simulink model "cnlib"  (Simulink 6.2)
settings: Solver=ode5  SolverMode=SingleTasking  StartTime=0.0  StopTime=5  FixedStep=0.001  MaxStep=0.001  RelTol=1e-3  AbsTol=1e-3
undefined symbols (not defined in the file): k
(part 1 of 7)
settings Model: Creator=jacobs  LastModifiedBy=jacobs  ExtModeAutoUpdateStatusClock=off
settings DataIOCC: LimitDataPoints=off  SaveOutput=off  SaveTime=off
settings OptimizationCC: BlockReduction=off  BooleanDataType=off
settings HardwareCC: TargetUnknown=on
settings STFCustomTargetCC: TargetFcnLib=ansi_tfl_tmw.mat  GenFloatMathFcnCalls=ANSI_C  ModelReferenceCompliant=off  SystemTargetFile=grt.tlc

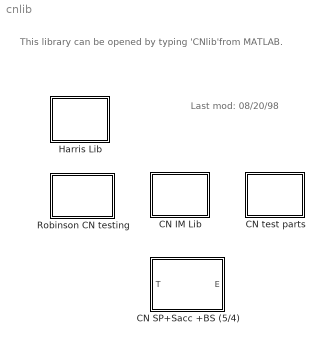
== system cnlib ==
  note: This library can be opened by typing
      |  'CNlib'from MATLAB.
  note: Last mod:
      | 08/20/98
  CN IM Lib : Subsystem
      mask Type: Lib
      mask Display: disp('CN IM\nLib')
  CN SP+Sacc +BS (5/4) : Subsystem
      mask init:
      | k=0.25;
      mask Display: disp('CN Model\nSP (DARm)\nSacc+BS')
  CN test parts : Subsystem
      mask Type: Lib
      mask Display: disp('CN Test\nParts')
  Harris Lib : Subsystem
      mask Display: disp('Harris\nLibrary')
  Robinson CN testing : Subsystem
      mask Display: disp('Robinson\nCN test')

== system cnlib/CN IM Lib ==
  BS Logic1 : Subsystem  Orientation=up
      mask Display: disp('BS/FS\nLogic')
  FS or BS? : Subsystem
      mask Display: disp('FS/BS?')
  IM (SP) 1z2p : Subsystem
      mask Display: disp('IM (SP)')
  IM (SP) 2p : Subsystem
      mask Display: disp('IM (SP)')
  IM (sacc) (FS) (old) : Subsystem
      mask Display: disp('IM (Sacc)')
  IM (sacc) (FS+BS) (old) : Subsystem
      mask Display: disp('IM (Sacc)')
  "IM (sacc) (FS+BS) (old) " : Subsystem
      mask Display: disp('IM (Sacc)')
  IM (sp) 1p : Subsystem
      mask Display: disp('IM (SP)')
  IM SP + Sacc (pos-vel) : Subsystem  Orientation=left
      mask Display: disp('IM\nSP + Sacc\n(pos-vel)')
  IM Sacc (pos-vel) (good!) : Subsystem
      mask Display: disp('IM\nSP + Sacc\n(pos-vel)')

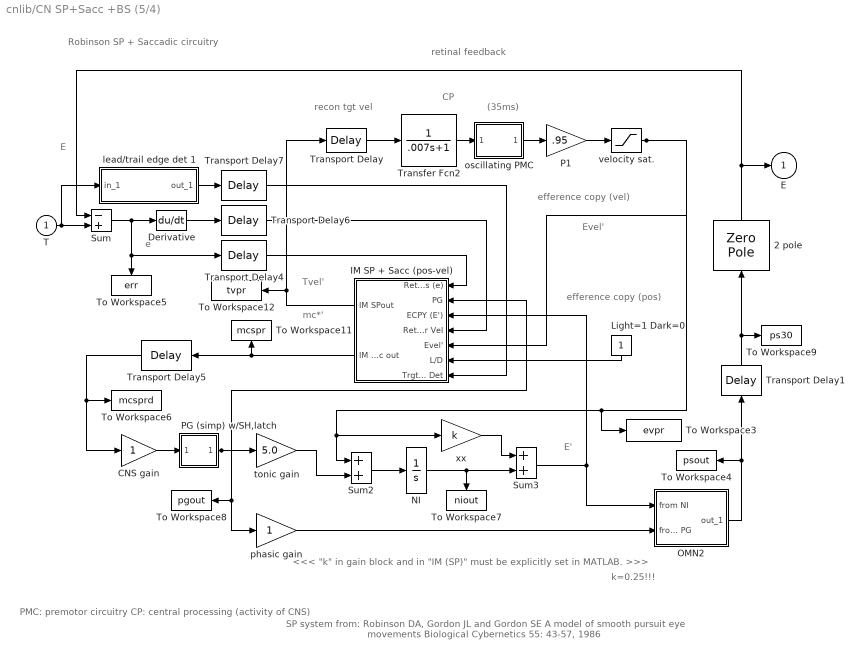
== system cnlib/CN SP+Sacc +BS (5/4) ==
  note: efference copy (pos)
  note: Evel'
  note: mc*'
  note: Tvel'
  note: e
  note: E
  note: E'
  note: k=0.25!!!
  note: retinal feedback
  note: recon tgt vel
  note: efference copy (vel)
  note: CP
  note: <<<  "k" in gain block and in "IM (SP)"
      | must be explicitly set in MATLAB.  >>>
  note: Robinson SP + Saccadic circuitry
  note: PMC: premotor circuitry
      | CP: central processing (activity of CNS)
  note: SP system from: Robinson DA, Gordon JL and Gordon SE
      | A model of smooth pursuit eye movements
      | Biological Cybernetics 55: 43-57,  1986
  note: (35ms)
  T : Inport  Port=1  LatchInput=off
  2 pole : ZeroPole  Orientation=up  Zeros=[ ]  Poles=[ -1/.18 -1/.007]  Gain=[1/.18 * 1/.007]
      mask Display: disp('2-pole\nPlant')
  CNS gain : Gain  SaturateOnIntegerOverflow=on
  Derivative : Derivative
      mask Display: disp('s')
  IM SP + Sacc (pos-vel) : Subsystem  Orientation=left
      mask Display: disp('IM\nSP + Sacc\n(pos-vel)')
  Light=1 Dark=0 : Constant  Orientation=down
  NI : Integrator
  OMN2 : Subsystem
      mask Display: disp('<--"tonic" \nOMN2\n<--"phasic"')
  P1 : Gain  Gain=.95  SaturateOnIntegerOverflow=on
  PG (simp) w/SH,latch : Subsystem
      mask Display: disp('PG')
  Sum : Sum  Inputs=-+  SaturateOnIntegerOverflow=on  InputSameDT=on
  Sum2 : Sum  SaturateOnIntegerOverflow=on  InputSameDT=on
  Sum3 : Sum  SaturateOnIntegerOverflow=on  InputSameDT=on
  To Workspace11 : ToWorkspace  VariableName=mcspr  SaveFormat=Array
      settings: Orientation=up  MaxDataPoints=10000
  To Workspace12 : ToWorkspace  VariableName=tvpr  SaveFormat=Array
      settings: MaxDataPoints=10000
  To Workspace3 : ToWorkspace  VariableName=evpr  SaveFormat=Array
      settings: MaxDataPoints=10000
  To Workspace4 : ToWorkspace  VariableName=psout  SaveFormat=Array
      settings: MaxDataPoints=10000
  To Workspace5 : ToWorkspace  VariableName=err  SaveFormat=Array
      settings: Orientation=down  MaxDataPoints=10000
  To Workspace6 : ToWorkspace  VariableName=mcsprd  SaveFormat=Array
      settings: MaxDataPoints=10000
  To Workspace7 : ToWorkspace  VariableName=niout  SaveFormat=Array
      settings: Orientation=down  MaxDataPoints=10000
  To Workspace8 : ToWorkspace  VariableName=pgout  SaveFormat=Array
      settings: MaxDataPoints=10000
  To Workspace9 : ToWorkspace  VariableName=ps30  SaveFormat=Array
      settings: MaxDataPoints=10000
  Transfer Fcn2 : TransferFcn  Denominator=[.007 1]
  Transport Delay : TransportDelay  DelayTime=0.015
      mask Display: disp('15ms')
  Transport Delay1 : TransportDelay  Orientation=up  DelayTime=0.03
      mask Display: disp('30ms')
  Transport Delay4 : TransportDelay  DelayTime=.05
      mask Display: disp('50ms')
  Transport Delay5 : TransportDelay  Orientation=left  DelayTime=0.001
      mask Display: disp('1ms')
  Transport Delay6 : TransportDelay  DelayTime=.05
      mask Display: disp('50ms')
  Transport Delay7 : TransportDelay  DelayTime=.05
      mask Display: disp('50ms')
  lead/trail edge det 1 : Subsystem
      mask Display: disp('Target Change\nDetection')
  oscillating PMC : Subsystem
      mask Display: disp('PMC+')
  phasic gain : Gain  SaturateOnIntegerOverflow=on
  tonic gain : Gain  Gain=5.0  SaturateOnIntegerOverflow=on
  velocity sat. : Saturate  UpperLimit=90  LowerLimit=-90
  xx : Gain  Gain=k  SaturateOnIntegerOverflow=on
  E : Outport  InitialOutput=0
  wires:
  Transport Delay5/1 -> CNS gain/1, To Workspace6/1
  CNS gain/1 -> PG (simp) w/SH,latch/1(in_1)
  PG (simp) w/SH,latch/1(out_1) -> phasic gain/1, To Workspace8/1, IM SP + Sacc (pos-vel)/2(PG), tonic gain/1
  IM SP + Sacc (pos-vel)/2(IM Sacc out) -> Transport Delay5/1, To Workspace11/1
  Transport Delay7/1 -> IM SP + Sacc (pos-vel)/7(TrgtChng Det)
  lead/trail edge det 1/1(out_1) -> Transport Delay7/1
  IM SP + Sacc (pos-vel)/1(IM SPout) -> Transport Delay/1, To Workspace12/1
  Derivative/1 -> Transport Delay6/1
  Transport Delay6/1 -> IM SP + Sacc (pos-vel)/4(RetErr Vel)
  Transport Delay1/1 -> 2 pole/1, To Workspace9/1
  Sum/1 -> Derivative/1, Transport Delay4/1, To Workspace5/1
  NI/1 -> Sum3/2, To Workspace7/1
  Sum3/1 -> IM SP + Sacc (pos-vel)/3(ECPY (E')), OMN2/1(from NI)
  velocity sat./1 -> IM SP + Sacc (pos-vel)/5(Evel'), Sum2/1, xx/1, To Workspace3/1
  Light=1 Dark=0/1 -> IM SP + Sacc (pos-vel)/6(L/D)
  xx/1 -> Sum3/1
  2 pole/1 -> E/1, Sum/1
  phasic gain/1 -> OMN2/2(from PG)
  OMN2/1(out_1) -> Transport Delay1/1, To Workspace4/1
  T/1 -> lead/trail edge det 1/1(in_1), Sum/2
  Sum2/1 -> NI/1
  tonic gain/1 -> Sum2/2
  Transfer Fcn2/1 -> oscillating PMC/1(desired eye vel)
  P1/1 -> velocity sat./1
  oscillating PMC/1(efference copy eye vel) -> P1/1
  Transport Delay/1 -> Transfer Fcn2/1
  Transport Delay4/1 -> IM SP + Sacc (pos-vel)/1(RetErr Pos (e))

== system cnlib/CN test parts ==
  Tgt moved? : Subsystem
      mask Display: disp('Tgt\nmoved?')
  mult sacc test : Subsystem
      mask Display: disp('mult\nsacc\ntest')
  summing test : Subsystem

== system cnlib/Harris Lib ==
  note: Harris Lib
  Harris Model : Subsystem
      mask Display: disp('Harris\n''95')

== system cnlib/Robinson CN testing ==
  note: Robinson Library (CN Testing)
  note: Last mod:
      | 08/20/98
  Robinson Fig. 8' : Subsystem
      mask Display: disp('Robinson\n(Osc.)')
  accel saturation : MATLABFcn  MATLABFcn=accsat
      mask Display: plot([-40 -8 8 40],[-120 -60 60 120], [0 0],[-120 120],[-40 40],[0 0])
  original PMC : Subsystem
      mask Display: disp('PMC')
  oscillating PMC : Subsystem
      mask Display: disp('PMC+')

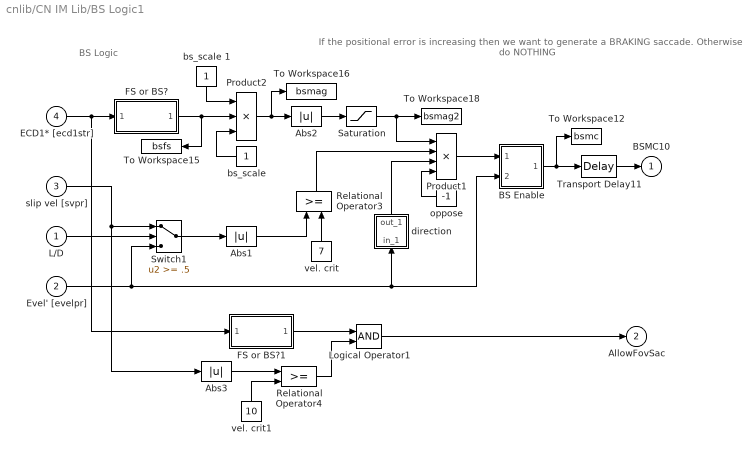
== system cnlib/CN IM Lib/BS Logic1 ==
  note: If the positional error is increasing then we want
      | to generate a BRAKING saccade.  Otherwise do NOTHING
  note: BS Logic
  L/D : Inport  Port=1  LatchInput=off
  Evel' [evelpr] : Inport  Port=2  LatchInput=off
  slip vel [svpr] : Inport  Port=3  LatchInput=off
  ECD1* [ecd1str] : Inport  Port=4  LatchInput=off
  Abs1 : Abs  SaturateOnIntegerOverflow=on
  Abs2 : Abs  SaturateOnIntegerOverflow=on
  Abs3 : Abs  SaturateOnIntegerOverflow=on
  BS Enable : Subsystem
      mask Display: disp('BS\nEnab')
  FS or BS? : Subsystem
      mask Display: disp('BS=1\nFS=0')
  FS or BS?1 : Subsystem
      mask Display: disp('FS=1\nBS=0')
  Logical Operator1 : Logic
  Product1 : Product  Inputs=4  SaturateOnIntegerOverflow=on  RndMeth=Zero  InputSameDT=on
  Product2 : Product  Inputs=3  SaturateOnIntegerOverflow=on  RndMeth=Zero  InputSameDT=on
  Relational Operator3 : RelationalOperator  Orientation=up  InputSameDT=on
  Relational Operator4 : RelationalOperator  InputSameDT=on
  Saturation : Saturate  UpperLimit=2  LowerLimit=0
  Switch1 : Switch  Threshold=.5  SaturateOnIntegerOverflow=on  InputSameDT=on
  To Workspace12 : ToWorkspace  VariableName=bsmc  SaveFormat=Array
      settings: MaxDataPoints=10000
  To Workspace15 : ToWorkspace  VariableName=bsfs  SaveFormat=Array
      settings: MaxDataPoints=10000
  To Workspace16 : ToWorkspace  VariableName=bsmag  SaveFormat=Array
      settings: MaxDataPoints=10000
  To Workspace18 : ToWorkspace  VariableName=bsmag2  SaveFormat=Array
      settings: MaxDataPoints=10000
  Transport Delay11 : TransportDelay  DelayTime=0.01
      mask Display: disp('10ms')
  "bs_scale " : Constant  Orientation=left
  bs_scale 1 : Constant  Orientation=down
  direction : Subsystem  Orientation=up
      mask Type: Sign
      mask Description: y = sign(x)
      mask Help: Sign Function:\n\t\t\ty = 1 if x > 0\n\t\t\ty = 0 if x = 0\n\t\t\ty = -1 if x < 0
      mask Display: plot(-50,-50,50,50,[-50,50],[0,0],[0,0],[-50,50],[-40,0],[-30,-30],[0,40],[30,30])
  oppose : Constant  Orientation=left  Value=-1
  vel. crit : Constant  Orientation=up  Value=7
  vel. crit1 : Constant  Orientation=up  Value=10
  BSMC10 : Outport  InitialOutput=0
  AllowFovSac : Outport  Port=2  InitialOutput=0
  wires:
  BS Enable/1("[bsmc]") -> To Workspace12/1, Transport Delay11/1
  Transport Delay11/1 -> BSMC10/1
  Relational Operator3/1 -> Product1/2
  direction/1(out_1) -> Product1/3
  oppose/1 -> Product1/4
  Product1/1 -> BS Enable/1("ecdiff1 ")
  Abs1/1 -> Relational Operator3/1
  vel. crit/1 -> Relational Operator3/2
  FS or BS?/1(BS=1 FS=0) -> To Workspace15/1, Product2/2
  L/D/1 -> Switch1/2
  Switch1/1 -> Abs1/1
  Abs2/1 -> Saturation/1
  Saturation/1 -> To Workspace18/1, Product1/1
  Product2/1 -> To Workspace16/1, Abs2/1
  "bs_scale "/1 -> Product2/3
  bs_scale 1/1 -> Product2/1
  ECD1* [ecd1str]/1 -> FS or BS?/1(pos error [ecd1str]), FS or BS?1/1(pos error [ecd1str])
  Evel' [evelpr]/1 -> direction/1(in_1), BS Enable/2("[evelpr]"), Switch1/3
  slip vel [svpr]/1 -> Switch1/1, Abs3/1
  Relational Operator4/1 -> Logical Operator1/2
  FS or BS?1/1(FS=1 BS=0) -> Logical Operator1/1
  Logical Operator1/1 -> AllowFovSac/1
  Abs3/1 -> Relational Operator4/1
  vel. crit1/1 -> Relational Operator4/2

== system cnlib/CN IM Lib/FS or BS? ==
  note: The position error is compared to its value 5 milliseconds earlier.
      | If the error is _increasing_, we want to make a braking
      | saccade to oppose the runaway.
  note: If the position error is _decreasing_, then the eye is approaching the
      | target, and we would like to generate a foveating saccade, since
      | this is our best time to consider capturing the target.
  note: FS or BS?
  pos error : Inport  Port=1  LatchInput=off
  Abs : Abs  SaturateOnIntegerOverflow=on
  Relational Operator : RelationalOperator  Operator=<=  InputSameDT=on
  Transport Delay1 : TransportDelay  DelayTime=.005
      mask Display: disp('5ms')
  FS or BS : Outport  InitialOutput=0
  wires:
  Transport Delay1/1 -> Relational Operator/2
  Relational Operator/1 -> FS or BS/1
  pos error/1 -> Abs/1
  Abs/1 -> Relational Operator/1, Transport Delay1/1

== system cnlib/CN IM Lib/IM (SP) 1z2p ==
  note: <<<  The "k" in gain and "Plant+ blocks"
      | must be explicitly set in MATLAB.  >>>
  note: IM (SP)
  in_1 : Inport  Port=1  LatchInput=off
  "\"Plant+\"" : ZeroPole  Zeros=[-1/k]  Poles=[ -1/.18 -1/.007]  Gain=[793.65*k]
  P2 : Gain  SaturateOnIntegerOverflow=on
  Transport Delay3 : TransportDelay  DelayTime=0.060
      mask Display: disp('60ms')
  out_1 : Outport  InitialOutput=0
  wires:
  Transport Delay3/1 -> out_1/1
  "\"Plant+\""/1 -> P2/1
  P2/1 -> Transport Delay3/1
  in_1/1 -> "\"Plant+\""/1

== system cnlib/CN IM Lib/IM (SP) 2p ==
  in_1 : Inport  Port=1  LatchInput=off
  P2 : Gain  SaturateOnIntegerOverflow=on
  "Robinson (142.8, 5.555)" : TransferFcn  Numerator=[1.0]  Denominator=[.00126 .187 1]
      mask Display: disp('2-pole\nPlant')
  Transport Delay3 : TransportDelay  DelayTime=0.08
      mask Display: disp('80ms')
  out_1 : Outport  InitialOutput=0
  wires:
  P2/1 -> Transport Delay3/1
  "Robinson (142.8, 5.555)"/1 -> P2/1
  in_1/1 -> "Robinson (142.8, 5.555)"/1
  Transport Delay3/1 -> out_1/1

== system cnlib/CN IM Lib/IM (sacc) (FS) (old) ==
  note: NOTE: so far, this block is only for FOVEATING
      | saccades.  The output is either zero, or the
      | retinal error (which is already the input to the PG).
  note: ((Note: the PG has its own built-in latency circuitry, so this probably
      | removes the need to add such functionality here.))
  note: For foveating saccades:
  note: Finally, we still must satisy the velocity criterion before we can generate
      |  a saccade.  Only if this condition is met, the pulse generator will
      | get the information needed to attempt to reduce the position error.
  note: This value is then compared to the threshold that must be exceeded
      | to generate a saccade.  If the value is greater than threshold it will be
      | passed along towards the output.  If not, the output will be zero.
  note: If Input 3 is '1' (light), then the efference copy of position (input 2)  is
      | passed to the rest of the block, otherwise an internal representation is used.
  note: Internal Monitor (sacc)
  note: Input 1: retinal error
      | Input 2: efference copy (pos)
      | Input 3: Light=1, dark = 0
      | Input 4: reconstructed tgt vel
      | Input 5: efference copy (vel)
  _ret err : Inport  Port=1  LatchInput=off
  _ec (pos) : Inport  Port=2  LatchInput=off
  _L/D? : Inport  Port=3  LatchInput=off
  _recon tgt vel : Inport  Port=4  LatchInput=off
  _ec (vel) : Inport  Port=5  LatchInput=off
  Logical Operator : Logic
  Product : Product  SaturateOnIntegerOverflow=on  RndMeth=Zero  InputSameDT=on
  Relational Operator : RelationalOperator  InputSameDT=on
  Relational Operator1 : RelationalOperator  InputSameDT=on
  Sum : Sum  SaturateOnIntegerOverflow=on  InputSameDT=on
  Switch1 : Switch  Threshold=.5  SaturateOnIntegerOverflow=on  InputSameDT=on
  Switch2 : Switch  Threshold=.5  SaturateOnIntegerOverflow=on  InputSameDT=on
  Transport Delay3 : TransportDelay  DelayTime=0.08
      mask Display: disp('80ms')
  pos (deg) criterion : Constant  Value=.1
  slip vel : Sum  Inputs=+-  SaturateOnIntegerOverflow=on  InputSameDT=on
  tgt pos (imag) : Constant  Value=0
  vel.(deg/sec) criterion : Constant  Orientation=up  Value=4
  out_1 : Outport  InitialOutput=0
  wires:
  _ec (vel)/1 -> Switch1/3, slip vel/2
  _L/D?/1 -> Switch1/2, Switch2/2
  Sum/1 -> Switch2/3
  tgt pos (imag)/1 -> Sum/2
  _ec (pos)/1 -> Sum/1
  _ret err/1 -> Switch2/1
  Switch2/1 -> Relational Operator/1, Product/1
  Product/1 -> Transport Delay3/1
  pos (deg) criterion/1 -> Relational Operator/2
  Transport Delay3/1 -> out_1/1
  Logical Operator/1 -> Product/2
  Relational Operator/1 -> Logical Operator/1
  slip vel/1 -> Switch1/1
  Switch1/1 -> Relational Operator1/1
  vel.(deg/sec) criterion/1 -> Relational Operator1/2
  Relational Operator1/1 -> Logical Operator/2
  _recon tgt vel/1 -> slip vel/1

== system cnlib/CN IM Lib/IM (sacc) (FS+BS) (old) ==
  note: Internal Monitor (sacc)
  note: Input 1: retinal error
      | Input 2: efference copy (pos)
      | Input 3: Light=1, dark = 0
      | Input 4: reconstructed tgt vel
      | Input 5: efference copy (vel)
  note: For foveating saccades: If Input 3 is '1' (light), then the
      | efference copy of position (input 2) is passed to the rest
      | of the block, otherwise an internal representation is used.
  note: This value is then compared to the threshold that must be
      | exceeded to generate a saccade.  If the value is greater
      | than threshold it will be passed along towards the output.
      | If not, the output will be zero.
  note: Finally, we still must satisy the velocity criterion before we
      | can generate  a saccade.  Only if this condition is met,
      | will the pulse generator get the information needed to
      | attempt to reduce the position error.
  note: ((Note: the PG has its own built-in latency circuitry, so this
      | probably removes the need to add such functionality here.))
  note: If the error is DECREASING, then we want to
      | generate a foveating saccade sufficient to
      | reduce the position error close to zero.
  note: For braking saccades: The position error
      | (retinal or imagined) is compared by "FS/BS"
      |  against its value 5ms earlier.  If the error is
      | INCREASING then we want to generate a
      | braking saccade of stereotyped magnitude
      | (presently 0.5 deg).
  note: ((We could also generate a RANDOM magnitude
      | braking saccade [0.1 .. 1.0] if we want))
  _ret err : Inport  Port=1  LatchInput=off
  _ec (pos) : Inport  Port=2  LatchInput=off
  _L/D? : Inport  Port=3  LatchInput=off
  _recon tgt vel : Inport  Port=4  LatchInput=off
  _ec (vel) : Inport  Port=5  LatchInput=off
  BS mag. : Constant  Orientation=up  Value=.5
  FS or BS? : Subsystem
      mask Display: disp('FS/BS?')
  Logical Operator : Logic
  Product : Product  SaturateOnIntegerOverflow=on  RndMeth=Zero  InputSameDT=on
  Relational Operator : RelationalOperator  InputSameDT=on
  Relational Operator1 : RelationalOperator  InputSameDT=on
  Sum : Sum  SaturateOnIntegerOverflow=on  InputSameDT=on
  Switch1 : Switch  Threshold=.5  SaturateOnIntegerOverflow=on  InputSameDT=on
  Switch2 : Switch  Threshold=.5  SaturateOnIntegerOverflow=on  InputSameDT=on
  Switch3 : Switch  Threshold=.5  SaturateOnIntegerOverflow=on  InputSameDT=on
  pos (deg) criterion : Constant  Value=.1
  slip vel : Sum  Inputs=+-  SaturateOnIntegerOverflow=on  InputSameDT=on
  tgt pos (imag) : Constant  Value=0
  vel.(deg/sec) criterion : Constant  Orientation=up  Value=4
  out_1 : Outport  InitialOutput=0
  wires:
  _recon tgt vel/1 -> slip vel/1
  Relational Operator1/1 -> Logical Operator/2
  vel.(deg/sec) criterion/1 -> Relational Operator1/2
  Switch1/1 -> Relational Operator1/1
  slip vel/1 -> Switch1/1
  Relational Operator/1 -> Logical Operator/1
  Logical Operator/1 -> Product/2
  pos (deg) criterion/1 -> Relational Operator/2
  _ret err/1 -> Switch2/1
  _ec (pos)/1 -> Sum/1
  tgt pos (imag)/1 -> Sum/2
  Sum/1 -> Switch2/3
  _ec (vel)/1 -> Switch1/3, slip vel/2
  _L/D?/1 -> Switch2/2, Switch1/2
  Switch3/1 -> out_1/1
  Product/1 -> Switch3/1
  BS mag./1 -> Switch3/3
  FS or BS?/1(FS or BS) -> Switch3/2
  Switch2/1 -> Relational Operator/1, Product/1, FS or BS?/1(pos error)

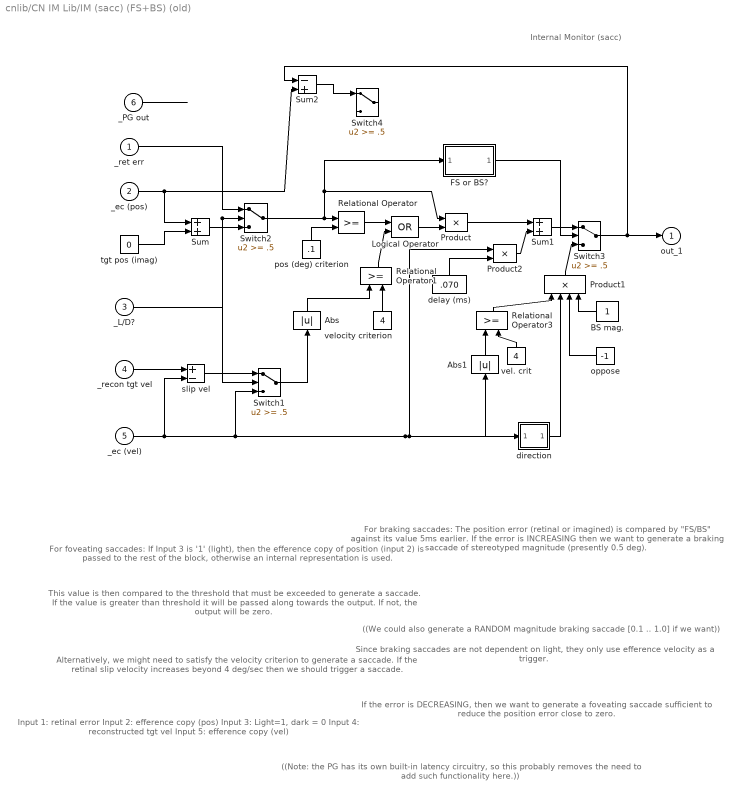
== system cnlib/CN IM Lib/IM (sacc) (FS+BS) (old)  ==
  note: For foveating saccades: If Input 3 is '1' (light), then the
      | efference copy of position (input 2) is passed to the rest
      | of the block, otherwise an internal representation is used.
  note: This value is then compared to the threshold that must be
      | exceeded to generate a saccade.  If the value is greater
      | than threshold it will be passed along towards the output.
      | If not, the output will be zero.
  note: Alternatively, we might need to satisfy the velocity criterion
      | to generate a saccade.  If the retinal slip velocity increases
      | beyond 4 deg/sec then we should trigger a saccade.
  note: For braking saccades: The position error
      | (retinal or imagined) is compared by "FS/BS"
      |  against its value 5ms earlier.  If the error is
      | INCREASING then we want to generate a
      | braking saccade of stereotyped magnitude
      | (presently 0.5 deg).
  note: ((We could also generate a RANDOM magnitude
      | braking saccade [0.1 .. 1.0] if we want))
  note: Input 1: retinal error
      | Input 2: efference copy (pos)
      | Input 3: Light=1, dark = 0
      | Input 4: reconstructed tgt vel
      | Input 5: efference copy (vel)
  note: ((Note: the PG has its own built-in latency circuitry, so this
      | probably removes the need to add such functionality here.))
  note: If the error is DECREASING, then we want to
      | generate a foveating saccade sufficient to
      | reduce the position error close to zero.
  note: Since braking saccades are not dependent on
      | light, they only use efference velocity as a trigger.
  note: Internal Monitor (sacc)
  _ret err : Inport  Port=1  LatchInput=off
  _ec (pos) : Inport  Port=2  LatchInput=off
  _L/D? : Inport  Port=3  LatchInput=off
  _recon tgt vel : Inport  Port=4  LatchInput=off
  _ec (vel) : Inport  Port=5  LatchInput=off
  _PG out : Inport  Port=6  LatchInput=off
  Abs : Abs  Orientation=up  SaturateOnIntegerOverflow=on
  Abs1 : Abs  Orientation=up  SaturateOnIntegerOverflow=on
  BS mag. : Constant  Orientation=left
  FS or BS? : Subsystem
      mask Display: disp('FS/BS?')
  Logical Operator : Logic  Operator=OR
  Product : Product  SaturateOnIntegerOverflow=on  RndMeth=Zero  InputSameDT=on
  Product1 : Product  Orientation=up  Inputs=4  SaturateOnIntegerOverflow=on  RndMeth=Zero  InputSameDT=on
  Product2 : Product  SaturateOnIntegerOverflow=on  RndMeth=Zero  InputSameDT=on
  Relational Operator : RelationalOperator  InputSameDT=on
  Relational Operator1 : RelationalOperator  Orientation=up  InputSameDT=on
  Relational Operator3 : RelationalOperator  Orientation=up  InputSameDT=on
  Sum : Sum  SaturateOnIntegerOverflow=on  InputSameDT=on
  Sum1 : Sum  SaturateOnIntegerOverflow=on  InputSameDT=on
  Sum2 : Sum  Inputs=-+  SaturateOnIntegerOverflow=on  InputSameDT=on
  Switch{1..4} (4 alike) : Switch  Threshold=.5  SaturateOnIntegerOverflow=on  InputSameDT=on
  delay (ms) : Constant  Orientation=up  Value=.070
  direction : Subsystem
      mask Type: Sign
      mask Description: y = sign(x)
      mask Help: Sign Function:\n\t\t\ty = 1 if x > 0\n\t\t\ty = 0 if x = 0\n\t\t\ty = -1 if x < 0
      mask Display: plot(-50,-50,50,50,[-50,50],[0,0],[0,0],[-50,50],[-40,0],[-30,-30],[0,40],[30,30])
  oppose : Constant  Orientation=left  Value=-1
  pos (deg) criterion : Constant  Orientation=up  Value=.1
  slip vel : Sum  Inputs=+-  SaturateOnIntegerOverflow=on  InputSameDT=on
  tgt pos (imag) : Constant  Value=0
  vel. crit : Constant  Orientation=up  Value=4
  velocity criterion : Constant  Orientation=up  Value=4
  out_1 : Outport  InitialOutput=0
  wires:
  _recon tgt vel/1 -> slip vel/1
  Relational Operator1/1 -> Logical Operator/2
  velocity criterion/1 -> Relational Operator1/2
  slip vel/1 -> Switch1/1
  Relational Operator/1 -> Logical Operator/1
  Logical Operator/1 -> Product/2
  pos (deg) criterion/1 -> Relational Operator/2
  _ret err/1 -> Switch2/1
  tgt pos (imag)/1 -> Sum/2
  Sum/1 -> Switch2/3
  FS or BS?/1(FS or BS) -> Switch3/2
  Relational Operator3/1 -> Product1/1
  Product1/1 -> Switch3/3
  Abs/1 -> Relational Operator1/1
  Switch1/1 -> Abs/1
  Abs1/1 -> Relational Operator3/1
  direction/1(out_1) -> Product1/2
  oppose/1 -> Product1/3
  BS mag./1 -> Product1/4
  vel. crit/1 -> Relational Operator3/2
  Product/1 -> Sum1/1
  Sum1/1 -> Switch3/1
  Product2/1 -> Sum1/2
  delay (ms)/1 -> Product2/2
  _ec (vel)/1 -> Switch1/3, Abs1/1, direction/1(in_1), Product2/1, slip vel/2
  _L/D?/1 -> Switch2/2, Switch1/2
  _PG out/1 -> ?
  Switch2/1 -> Relational Operator/1, Product/1, FS or BS?/1(pos error)
  Switch3/1 -> out_1/1, Sum2/1
  _ec (pos)/1 -> Sum/1, Sum2/2
  ? -> Switch4/2
  Sum2/1 -> Switch4/1

== system cnlib/CN IM Lib/IM (sp) 1p ==
  in_1 : Inport  Port=1  LatchInput=off
  "\"plant\"" : TransferFcn  Denominator=[0.015 1]
  P2 : Gain  SaturateOnIntegerOverflow=on
  Transport Delay3 : TransportDelay  DelayTime=0.08
      mask Display: disp('80ms')
  out_1 : Outport  InitialOutput=0
  wires:
  Transport Delay3/1 -> out_1/1
  in_1/1 -> "\"plant\""/1
  "\"plant\""/1 -> P2/1
  P2/1 -> Transport Delay3/1

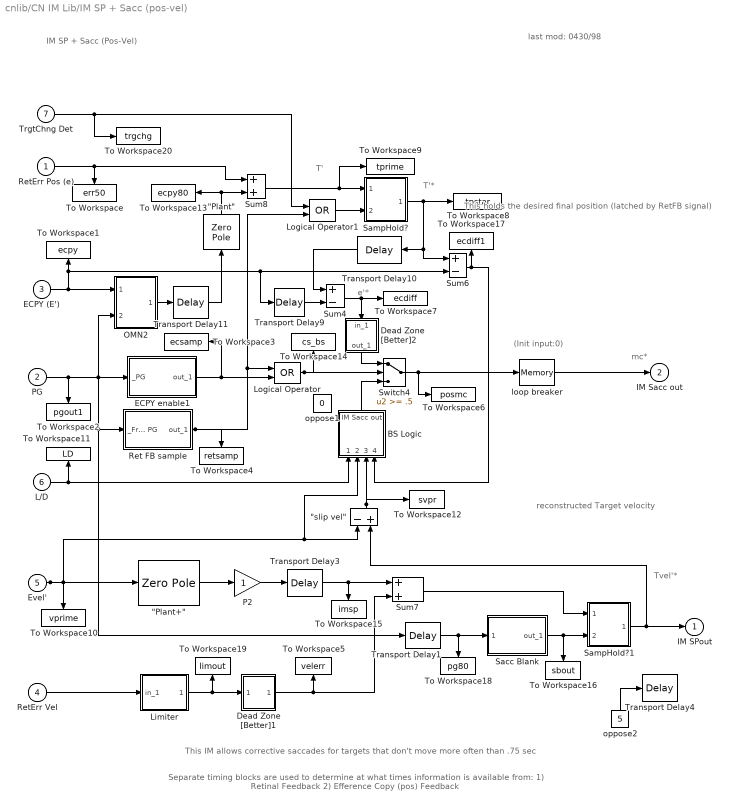
== system cnlib/CN IM Lib/IM SP + Sacc (pos-vel) ==
  note: T'
  note: e'*
  note: Tvel'*
  note: mc*
  note: T'*
  note: last mod:
      | 0430/98
  note: IM SP + Sacc (Pos-Vel)
  note: This holds the desired final position
      | (latched by RetFB signal)
  note: reconstructed Target velocity
  note: This IM allows corrective saccades for targets that don't move more often than .75 sec
  note: Separate timing blocks are used to determine at what times information is available from:
      | 1) Retinal Feedback
      | 2) Efference Copy (pos) Feedback
  note: (Init input:0)
  RetErr Pos (e) : Inport  Port=1  LatchInput=off
  PG : Inport  Port=2  LatchInput=off
  ECPY (E') : Inport  Port=3  LatchInput=off
  RetErr Vel : Inport  Port=4  LatchInput=off
  Evel' : Inport  Port=5  LatchInput=off
  L/D : Inport  Port=6  LatchInput=off
  TrgtChng Det : Inport  Port=7  LatchInput=off
  "\"Plant\"" : ZeroPole  Orientation=up  Zeros=[ ]  Poles=[ -1/.18 -1/.007]  Gain=[1/.18 * 1/.007]
      mask Display: disp('2-pole\nPlant')
  "\"Plant+\"" : ZeroPole  Zeros=[-1/k]  Poles=[ -1/.18 -1/.007]  Gain=[793.65*k]
      mask Display: disp('1-zero\n2pole\n"Plant+"')
  "\"slip vel\"" : Sum  Orientation=up  Inputs=-+  SaturateOnIntegerOverflow=on  InputSameDT=on
  BS Logic : Subsystem  Orientation=up
      mask Display: disp('BS\nLogic')
  Dead Zone [Better]1 : Subsystem
      mask Display: disp('Dead\nZone')
  Dead Zone [Better]2 : Subsystem  Orientation=down
      mask Display: disp('Dead\nZone')
  ECPY enable1 : Subsystem
      mask Display: disp('ECPY\nEnable')
  Limiter : Subsystem
      mask Display: disp('Limiter')
  Logical Operator : Logic  Operator=OR
  Logical Operator1 : Logic  Operator=OR
  OMN2 : Subsystem
      mask Display: disp('<--"t" \nOMN2\n<--"ph"')
  P2 : Gain  SaturateOnIntegerOverflow=on
  Ret FB sample : Subsystem
      mask Display: disp('Ret FB\nEnable')
  Sacc Blank : Subsystem
      mask Display: disp('Saccade\nBlanking')
  SampHold? : Subsystem
      mask Display: disp('S&H\n(S=H)\n(H=L)')
  SampHold?1 : Subsystem
      mask Display: disp('S&H\n(S=H)\n(H=L)')
  Sum4 : Sum  Inputs=+-  SaturateOnIntegerOverflow=on  InputSameDT=on
  Sum6 : Sum  Inputs=+-  SaturateOnIntegerOverflow=on  InputSameDT=on
  Sum7 : Sum  SaturateOnIntegerOverflow=on  InputSameDT=on
  Sum8 : Sum  SaturateOnIntegerOverflow=on  InputSameDT=on
  Switch4 : Switch  Threshold=.5  SaturateOnIntegerOverflow=on  InputSameDT=on
  To Workspace : ToWorkspace  VariableName=err50  SaveFormat=Array
      settings: Orientation=down  MaxDataPoints=10000
  To Workspace1 : ToWorkspace  VariableName=ecpy  SaveFormat=Array
      settings: Orientation=up  MaxDataPoints=10000
  To Workspace10 : ToWorkspace  VariableName=vprime  SaveFormat=Array
      settings: Orientation=down  MaxDataPoints=10000
  To Workspace11 : ToWorkspace  VariableName=LD  SaveFormat=Array
      settings: Orientation=up  MaxDataPoints=10000
  To Workspace12 : ToWorkspace  VariableName=svpr  SaveFormat=Array
      settings: MaxDataPoints=10000
  To Workspace13 : ToWorkspace  VariableName=ecpy80  SaveFormat=Array
      settings: MaxDataPoints=10000
  To Workspace14 : ToWorkspace  VariableName=cs_bs  SaveFormat=Array
      settings: Orientation=up  MaxDataPoints=10000
      mask Type: imsw1in
  To Workspace15 : ToWorkspace  VariableName=imsp  SaveFormat=Array
      settings: Orientation=down  MaxDataPoints=10000
  To Workspace16 : ToWorkspace  VariableName=sbout  SaveFormat=Array
      settings: Orientation=down  MaxDataPoints=10000
  To Workspace17 : ToWorkspace  VariableName=ecdiff1  SaveFormat=Array
      settings: Orientation=up  MaxDataPoints=10000
  To Workspace18 : ToWorkspace  VariableName=pg80  SaveFormat=Array
      settings: Orientation=down  MaxDataPoints=10000
  To Workspace19 : ToWorkspace  VariableName=limout  SaveFormat=Array
      settings: Orientation=up  MaxDataPoints=10000
  To Workspace2 : ToWorkspace  VariableName=pgout1  SaveFormat=Array
      settings: Orientation=down  MaxDataPoints=10000
  To Workspace20 : ToWorkspace  VariableName=trgchg  SaveFormat=Array
      settings: MaxDataPoints=10000
  To Workspace3 : ToWorkspace  VariableName=ecsamp  SaveFormat=Array
      settings: MaxDataPoints=10000
      mask Type: imsw1in
  To Workspace4 : ToWorkspace  VariableName=retsamp  SaveFormat=Array
      settings: Orientation=down  MaxDataPoints=10000
      mask Type: imsw1in
  To Workspace5 : ToWorkspace  VariableName=velerr  SaveFormat=Array
      settings: Orientation=up  MaxDataPoints=10000
  To Workspace6 : ToWorkspace  VariableName=posmc  SaveFormat=Array
      settings: MaxDataPoints=10000
  To Workspace7 : ToWorkspace  VariableName=ecdiff  SaveFormat=Array
      settings: MaxDataPoints=10000
  To Workspace8 : ToWorkspace  VariableName=tpstar  SaveFormat=Array
      settings: MaxDataPoints=10000
  To Workspace9 : ToWorkspace  VariableName=tprime  SaveFormat=Array
      settings: MaxDataPoints=10000
  Transport Delay1 : TransportDelay  DelayTime=0.080
      mask Display: disp('80ms')
  Transport Delay10 : TransportDelay  Orientation=left  DelayTime=.12
      mask Display: disp('120ms')
  Transport Delay11 : TransportDelay  DelayTime=0.080
      mask Display: disp('80ms')
  Transport Delay3 : TransportDelay  DelayTime=0.08
      mask Display: disp('80ms')
  Transport Delay4 : TransportDelay  DelayTime=0.05
      mask Display: disp('50ms')
  Transport Delay9 : TransportDelay  DelayTime=.05
      mask Display: disp('50ms')
  loop breaker : Memory
  oppose1 : Constant  Orientation=up  Value=0
  oppose2 : Constant  Orientation=up  Value=5
  IM SPout : Outport  InitialOutput=0
  IM Sacc out : Outport  Port=2  InitialOutput=0
  wires:
  loop breaker/1 -> IM Sacc out/1
  Transport Delay9/1 -> Sum4/2
  Transport Delay10/1 -> Sum4/1
  ECPY (E')/1 -> OMN2/1(from NI), Transport Delay9/1, Sum6/2, To Workspace1/1
  Sum6/1 -> To Workspace17/1, BS Logic/4(ECdiff1)
  Switch4/1 -> To Workspace6/1, loop breaker/1
  Ret FB sample/1(out_1) -> To Workspace4/1, Logical Operator/1, Logical Operator1/2
  P2/1 -> Transport Delay3/1
  "\"Plant+\""/1 -> P2/1
  Evel'/1 -> "\"Plant+\""/1, BS Logic/2(Evel'), "\"slip vel\""/1, To Workspace10/1
  RetErr Vel/1 -> Limiter/1(in_1)
  "\"slip vel\""/1 -> BS Logic/3(slip vel), To Workspace12/1
  Logical Operator/1 -> To Workspace14/1, Switch4/2
  L/D/1 -> To Workspace11/1, BS Logic/1(L/D)
  PG/1 -> To Workspace2/1, OMN2/2(from PG), Ret FB sample/1(_From PG), Transport Delay1/1, ECPY enable1/1(_PG)
  Limiter/1(out_1) -> To Workspace19/1, Dead Zone [Better]1/1(in_1)
  ECPY enable1/1(out_1) -> To Workspace3/1, Logical Operator/2
  Sum4/1 -> Dead Zone [Better]2/1(in_1), To Workspace7/1
  Dead Zone [Better]2/1(out_1) -> Switch4/1
  Sum8/1 -> To Workspace9/1, SampHold?/1(Input)
  OMN2/1(out_1) -> Transport Delay11/1
  SampHold?/1(output) -> Sum6/1, Transport Delay10/1, To Workspace8/1
  Logical Operator1/1 -> SampHold?/2(S/H?)
  TrgtChng Det/1 -> To Workspace20/1, Logical Operator1/1
  "\"Plant\""/1 -> To Workspace13/1, Sum8/2
  RetErr Pos (e)/1 -> Sum8/1, To Workspace/1
  Transport Delay11/1 -> "\"Plant\""/1
  oppose2/1 -> Transport Delay4/1
  Transport Delay3/1 -> To Workspace15/1, Sum7/1
  Dead Zone [Better]1/1(out_1) -> To Workspace5/1, Sum7/2
  Transport Delay1/1 -> Sacc Blank/1(_From PG), To Workspace18/1
  Sacc Blank/1(out_1) -> To Workspace16/1, SampHold?1/2(S/H?)
  Sum7/1 -> SampHold?1/1(Input)
  SampHold?1/1(output) -> "\"slip vel\""/2, IM SPout/1
  BS Logic/1(IM Sacc out) -> Switch4/3

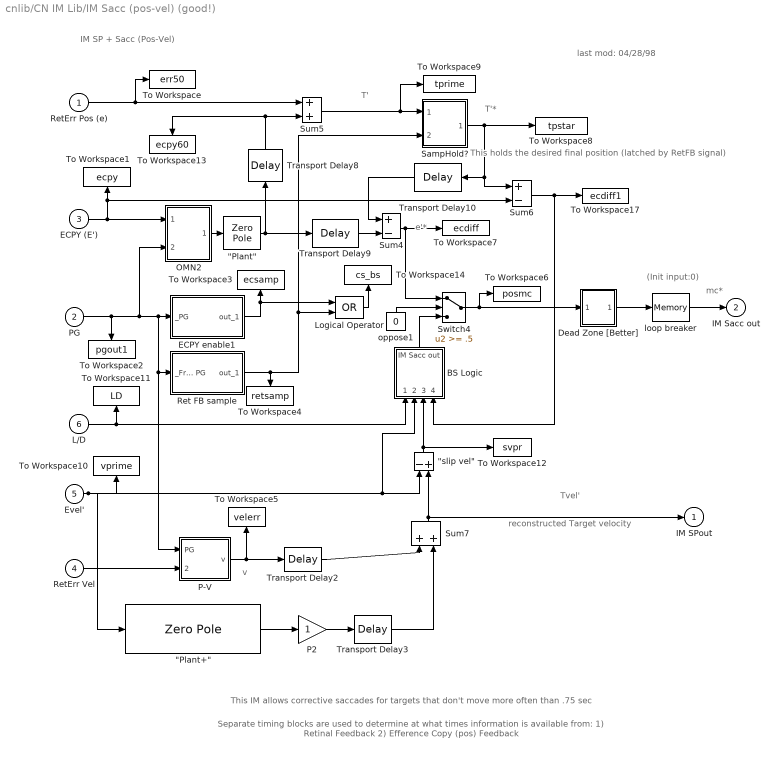
== system cnlib/CN IM Lib/IM Sacc (pos-vel) (good!) ==
  note: IM SP + Sacc (Pos-Vel)
  note: last mod:
      | 04/28/98
  note: T'*
  note: This holds the desired final position
      | (latched by RetFB signal)
  note: mc*
  note: T'
  note: (Init input:0)
  note: Tvel'
  note: This IM allows corrective saccades for targets that don't move more often than .75 sec
  note: Separate timing blocks are used to determine at what times information is available from:
      | 1) Retinal Feedback
      | 2) Efference Copy (pos) Feedback
  note: v
  note: e'*
  note: reconstructed Target velocity
  RetErr Pos (e) : Inport  Port=1  LatchInput=off
  PG : Inport  Port=2  LatchInput=off
  ECPY (E') : Inport  Port=3  LatchInput=off
  RetErr Vel : Inport  Port=4  LatchInput=off
  Evel' : Inport  Port=5  LatchInput=off
  L/D : Inport  Port=6  LatchInput=off
  "\"Plant\"" : ZeroPole  Zeros=[ ]  Poles=[ -1/.18 -1/.007]  Gain=[1/.18 * 1/.007]
      mask Display: disp('2-pole\nPlant')
  "\"Plant+\"" : ZeroPole  Zeros=[-1/k]  Poles=[ -1/.18 -1/.007]  Gain=[793.65*k]
      mask Display: disp('1-zero\n2pole\n"Plant+"')
  "\"slip vel\"" : Sum  Orientation=up  Inputs=-+  SaturateOnIntegerOverflow=on  InputSameDT=on
  BS Logic : Subsystem  Orientation=up
      mask Display: disp('BS\nLogic')
  Dead Zone [Better] : Subsystem
      mask Display: disp('Dead\nZone')
  ECPY enable1 : Subsystem
      mask Display: disp('ECPY\nEnable')
  Logical Operator : Logic  Operator=OR
  OMN2 : Subsystem
      mask Display: disp('<--"t" \nOMN2\n<--"ph"')
  P-V : Subsystem
      mask Display: disp('Smooth\nVelocity')
  P2 : Gain  SaturateOnIntegerOverflow=on
  Ret FB sample : Subsystem
      mask Display: disp('Ret FB\nEnable')
  SampHold? : Subsystem
      mask Display: disp('S&H\n(S=H)\n(H=L)')
  Sum4 : Sum  Inputs=+-  SaturateOnIntegerOverflow=on  InputSameDT=on
  Sum5 : Sum  SaturateOnIntegerOverflow=on  InputSameDT=on
  Sum6 : Sum  Inputs=+-  SaturateOnIntegerOverflow=on  InputSameDT=on
  Sum7 : Sum  Orientation=up  SaturateOnIntegerOverflow=on  InputSameDT=on
  Switch4 : Switch  Threshold=.5  SaturateOnIntegerOverflow=on  InputSameDT=on
  To Workspace : ToWorkspace  VariableName=err50  SaveFormat=Array
      settings: MaxDataPoints=10000
  To Workspace1 : ToWorkspace  VariableName=ecpy  SaveFormat=Array
      settings: Orientation=up  MaxDataPoints=10000
  To Workspace10 : ToWorkspace  VariableName=vprime  SaveFormat=Array
      settings: Orientation=up  MaxDataPoints=10000
  To Workspace11 : ToWorkspace  VariableName=LD  SaveFormat=Array
      settings: Orientation=up  MaxDataPoints=10000
  To Workspace12 : ToWorkspace  VariableName=svpr  SaveFormat=Array
      settings: MaxDataPoints=10000
  To Workspace13 : ToWorkspace  VariableName=ecpy60  SaveFormat=Array
      settings: Orientation=down  MaxDataPoints=10000
  To Workspace14 : ToWorkspace  VariableName=cs_bs  SaveFormat=Array
      settings: Orientation=up  MaxDataPoints=10000
      mask Type: imsw1in
  To Workspace17 : ToWorkspace  VariableName=ecdiff1  SaveFormat=Array
      settings: MaxDataPoints=10000
  To Workspace2 : ToWorkspace  VariableName=pgout1  SaveFormat=Array
      settings: Orientation=down  MaxDataPoints=10000
  To Workspace3 : ToWorkspace  VariableName=ecsamp  SaveFormat=Array
      settings: Orientation=up  MaxDataPoints=10000
      mask Type: imsw1in
  To Workspace4 : ToWorkspace  VariableName=retsamp  SaveFormat=Array
      settings: Orientation=down  MaxDataPoints=10000
      mask Type: imsw1in
  To Workspace5 : ToWorkspace  VariableName=velerr  SaveFormat=Array
      settings: Orientation=up  MaxDataPoints=10000
  To Workspace6 : ToWorkspace  VariableName=posmc  SaveFormat=Array
      settings: MaxDataPoints=10000
  To Workspace7 : ToWorkspace  VariableName=ecdiff  SaveFormat=Array
      settings: MaxDataPoints=10000
  To Workspace8 : ToWorkspace  VariableName=tpstar  SaveFormat=Array
      settings: MaxDataPoints=10000
  To Workspace9 : ToWorkspace  VariableName=tprime  SaveFormat=Array
      settings: MaxDataPoints=10000
  Transport Delay10 : TransportDelay  Orientation=left  DelayTime=.1
      mask Display: disp('100ms')
  Transport Delay2 : TransportDelay  DelayTime=0.03
      mask Display: disp('30ms')
  Transport Delay3 : TransportDelay  DelayTime=0.060
      mask Display: disp('60ms')
  Transport Delay8 : TransportDelay  Orientation=up  DelayTime=0.060
      mask Display: disp('60ms')
  Transport Delay9 : TransportDelay  DelayTime=.11
      mask Display: disp('110ms')
  loop breaker : Memory
  oppose1 : Constant  Orientation=up  Value=0
  IM SPout : Outport  InitialOutput=0
  IM Sacc out : Outport  Port=2  InitialOutput=0
  wires:
  loop breaker/1 -> IM Sacc out/1
  Transport Delay9/1 -> Sum4/2
  Sum4/1 -> To Workspace7/1, Switch4/1
  RetErr Pos (e)/1 -> Sum5/1, To Workspace/1
  Transport Delay10/1 -> Sum4/1
  "\"Plant\""/1 -> Transport Delay9/1, Transport Delay8/1
  SampHold?/1(output) -> To Workspace8/1, Transport Delay10/1, Sum6/1
  Transport Delay8/1 -> Sum5/2, To Workspace13/1
  OMN2/1(out_1) -> "\"Plant\""/1
  Dead Zone [Better]/1(out_1) -> loop breaker/1
  ECPY (E')/1 -> OMN2/1(from NI), To Workspace1/1, Sum6/2
  Logical Operator/1 -> To Workspace14/1
  Sum5/1 -> SampHold?/1(Input), To Workspace9/1
  Switch4/1 -> Dead Zone [Better]/1(in_1), To Workspace6/1
  Ret FB sample/1(out_1) -> To Workspace4/1, SampHold?/2(S/H?), Logical Operator/2
  P2/1 -> Transport Delay3/1
  "\"Plant+\""/1 -> P2/1
  Transport Delay2/1 -> Sum7/1
  Transport Delay3/1 -> Sum7/2
  P-V/1(v) -> Transport Delay2/1, To Workspace5/1
  PG/1 -> OMN2/2(from PG), ECPY enable1/1(_PG), P-V/1(PG), Ret FB sample/1(_From PG), To Workspace2/1
  BS Logic/1(IM Sacc out) -> Switch4/3
  Sum6/1 -> To Workspace17/1, BS Logic/4(ECdiff1)
  L/D/1 -> BS Logic/1(L/D), To Workspace11/1
  oppose1/1 -> Switch4/2
  ECPY enable1/1(out_1) -> Logical Operator/1, To Workspace3/1
  Evel'/1 -> "\"Plant+\""/1, To Workspace10/1, "\"slip vel\""/1, BS Logic/2(Evel')
  RetErr Vel/1 -> P-V/2(Ret Err (vel))
  "\"slip vel\""/1 -> BS Logic/3(slip vel), To Workspace12/1
  Sum7/1 -> "\"slip vel\""/2, IM SPout/1

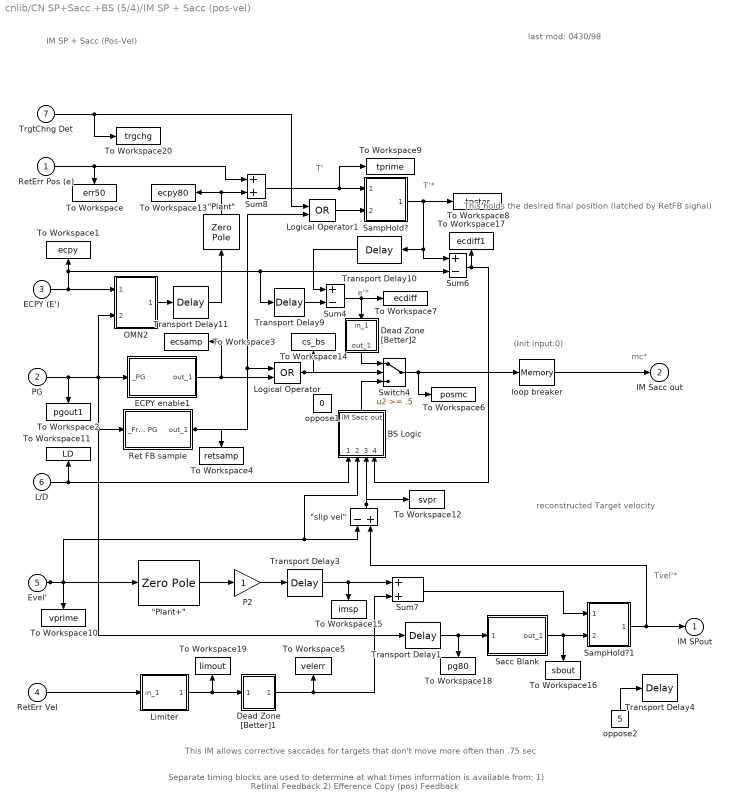
== system cnlib/CN SP+Sacc +BS (5/4)/IM SP + Sacc (pos-vel) ==
  note: (Init input:0)
  note: Separate timing blocks are used to determine at what times information is available from:
      | 1) Retinal Feedback
      | 2) Efference Copy (pos) Feedback
  note: This IM allows corrective saccades for targets that don't move more often than .75 sec
  note: reconstructed Target velocity
  note: This holds the desired final position
      | (latched by RetFB signal)
  note: IM SP + Sacc (Pos-Vel)
  note: last mod:
      | 0430/98
  note: T'*
  note: mc*
  note: Tvel'*
  note: e'*
  note: T'
  RetErr Pos (e) : Inport  Port=1  LatchInput=off
  PG : Inport  Port=2  LatchInput=off
  ECPY (E') : Inport  Port=3  LatchInput=off
  RetErr Vel : Inport  Port=4  LatchInput=off
  Evel' : Inport  Port=5  LatchInput=off
  L/D : Inport  Port=6  LatchInput=off
  TrgtChng Det : Inport  Port=7  LatchInput=off
  "\"Plant\"" : ZeroPole  Orientation=up  Zeros=[ ]  Poles=[ -1/.18 -1/.007]  Gain=[1/.18 * 1/.007]
      mask Display: disp('2-pole\nPlant')
  "\"Plant+\"" : ZeroPole  Zeros=[-1/k]  Poles=[ -1/.18 -1/.007]  Gain=[793.65*k]
      mask Display: disp('1-zero\n2pole\n"Plant+"')
  "\"slip vel\"" : Sum  Orientation=up  Inputs=-+  SaturateOnIntegerOverflow=on  InputSameDT=on
  BS Logic : Subsystem  Orientation=up
      mask Display: disp('BS\nLogic')
  Dead Zone [Better]1 : Subsystem
      mask Display: disp('Dead\nZone')
  Dead Zone [Better]2 : Subsystem  Orientation=down
      mask Display: disp('Dead\nZone')
  ECPY enable1 : Subsystem
      mask Display: disp('ECPY\nEnable')
  Limiter : Subsystem
      mask Display: disp('Limiter')
  Logical Operator : Logic  Operator=OR
  Logical Operator1 : Logic  Operator=OR
  OMN2 : Subsystem
      mask Display: disp('<--"t" \nOMN2\n<--"ph"')
  P2 : Gain  SaturateOnIntegerOverflow=on
  Ret FB sample : Subsystem
      mask Display: disp('Ret FB\nEnable')
  Sacc Blank : Subsystem
      mask Display: disp('Saccade\nBlanking')
  SampHold? : Subsystem
      mask Display: disp('S&H\n(S=H)\n(H=L)')
  SampHold?1 : Subsystem
      mask Display: disp('S&H\n(S=H)\n(H=L)')
  Sum4 : Sum  Inputs=+-  SaturateOnIntegerOverflow=on  InputSameDT=on
  Sum6 : Sum  Inputs=+-  SaturateOnIntegerOverflow=on  InputSameDT=on
  Sum7 : Sum  SaturateOnIntegerOverflow=on  InputSameDT=on
  Sum8 : Sum  SaturateOnIntegerOverflow=on  InputSameDT=on
  Switch4 : Switch  Threshold=.5  SaturateOnIntegerOverflow=on  InputSameDT=on
  To Workspace : ToWorkspace  VariableName=err50  SaveFormat=Array
      settings: Orientation=down  MaxDataPoints=10000
  To Workspace1 : ToWorkspace  VariableName=ecpy  SaveFormat=Array
      settings: Orientation=up  MaxDataPoints=10000
  To Workspace10 : ToWorkspace  VariableName=vprime  SaveFormat=Array
      settings: Orientation=down  MaxDataPoints=10000
  To Workspace11 : ToWorkspace  VariableName=LD  SaveFormat=Array
      settings: Orientation=up  MaxDataPoints=10000
  To Workspace12 : ToWorkspace  VariableName=svpr  SaveFormat=Array
      settings: MaxDataPoints=10000
  To Workspace13 : ToWorkspace  VariableName=ecpy80  SaveFormat=Array
      settings: MaxDataPoints=10000
  To Workspace14 : ToWorkspace  VariableName=cs_bs  SaveFormat=Array
      settings: Orientation=up  MaxDataPoints=10000
      mask Type: imsw1in
  To Workspace15 : ToWorkspace  VariableName=imsp  SaveFormat=Array
      settings: Orientation=down  MaxDataPoints=10000
  To Workspace16 : ToWorkspace  VariableName=sbout  SaveFormat=Array
      settings: Orientation=down  MaxDataPoints=10000
  To Workspace17 : ToWorkspace  VariableName=ecdiff1  SaveFormat=Array
      settings: Orientation=up  MaxDataPoints=10000
  To Workspace18 : ToWorkspace  VariableName=pg80  SaveFormat=Array
      settings: Orientation=down  MaxDataPoints=10000
  To Workspace19 : ToWorkspace  VariableName=limout  SaveFormat=Array
      settings: Orientation=up  MaxDataPoints=10000
  To Workspace2 : ToWorkspace  VariableName=pgout1  SaveFormat=Array
      settings: Orientation=down  MaxDataPoints=10000
  To Workspace20 : ToWorkspace  VariableName=trgchg  SaveFormat=Array
      settings: MaxDataPoints=10000
  To Workspace3 : ToWorkspace  VariableName=ecsamp  SaveFormat=Array
      settings: MaxDataPoints=10000
      mask Type: imsw1in
  To Workspace4 : ToWorkspace  VariableName=retsamp  SaveFormat=Array
      settings: Orientation=down  MaxDataPoints=10000
      mask Type: imsw1in
  To Workspace5 : ToWorkspace  VariableName=velerr  SaveFormat=Array
      settings: Orientation=up  MaxDataPoints=10000
  To Workspace6 : ToWorkspace  VariableName=posmc  SaveFormat=Array
      settings: MaxDataPoints=10000
  To Workspace7 : ToWorkspace  VariableName=ecdiff  SaveFormat=Array
      settings: MaxDataPoints=10000
  To Workspace8 : ToWorkspace  VariableName=tpstar  SaveFormat=Array
      settings: MaxDataPoints=10000
  To Workspace9 : ToWorkspace  VariableName=tprime  SaveFormat=Array
      settings: MaxDataPoints=10000
  Transport Delay1 : TransportDelay  DelayTime=0.080
      mask Display: disp('80ms')
  Transport Delay10 : TransportDelay  Orientation=left  DelayTime=.12
      mask Display: disp('120ms')
  Transport Delay11 : TransportDelay  DelayTime=0.080
      mask Display: disp('80ms')
  Transport Delay3 : TransportDelay  DelayTime=0.08
      mask Display: disp('80ms')
  Transport Delay4 : TransportDelay  DelayTime=0.05
      mask Display: disp('50ms')
  Transport Delay9 : TransportDelay  DelayTime=.05
      mask Display: disp('50ms')
  loop breaker : Memory
  oppose1 : Constant  Orientation=up  Value=0
  oppose2 : Constant  Orientation=up  Value=5
  IM SPout : Outport  InitialOutput=0
  IM Sacc out : Outport  Port=2  InitialOutput=0
  wires:
  BS Logic/1(IM Sacc out) -> Switch4/3
  SampHold?1/1(output) -> IM SPout/1, "\"slip vel\""/2
  Sum7/1 -> SampHold?1/1(Input)
  Sacc Blank/1(out_1) -> SampHold?1/2(S/H?), To Workspace16/1
  Transport Delay1/1 -> To Workspace18/1, Sacc Blank/1(_From PG)
  Dead Zone [Better]1/1(out_1) -> Sum7/2, To Workspace5/1
  Transport Delay3/1 -> Sum7/1, To Workspace15/1
  oppose2/1 -> Transport Delay4/1
  Transport Delay11/1 -> "\"Plant\""/1
  RetErr Pos (e)/1 -> To Workspace/1, Sum8/1
  "\"Plant\""/1 -> Sum8/2, To Workspace13/1
  TrgtChng Det/1 -> Logical Operator1/1, To Workspace20/1
  Logical Operator1/1 -> SampHold?/2(S/H?)
  SampHold?/1(output) -> To Workspace8/1, Transport Delay10/1, Sum6/1
  OMN2/1(out_1) -> Transport Delay11/1
  Sum8/1 -> SampHold?/1(Input), To Workspace9/1
  Dead Zone [Better]2/1(out_1) -> Switch4/1
  Sum4/1 -> To Workspace7/1, Dead Zone [Better]2/1(in_1)
  ECPY enable1/1(out_1) -> Logical Operator/2, To Workspace3/1
  Limiter/1(out_1) -> Dead Zone [Better]1/1(in_1), To Workspace19/1
  PG/1 -> ECPY enable1/1(_PG), Transport Delay1/1, Ret FB sample/1(_From PG), OMN2/2(from PG), To Workspace2/1
  L/D/1 -> BS Logic/1(L/D), To Workspace11/1
  Logical Operator/1 -> Switch4/2, To Workspace14/1
  "\"slip vel\""/1 -> To Workspace12/1, BS Logic/3(slip vel)
  RetErr Vel/1 -> Limiter/1(in_1)
  Evel'/1 -> To Workspace10/1, "\"slip vel\""/1, BS Logic/2(Evel'), "\"Plant+\""/1
  "\"Plant+\""/1 -> P2/1
  P2/1 -> Transport Delay3/1
  Ret FB sample/1(out_1) -> Logical Operator1/2, Logical Operator/1, To Workspace4/1
  Switch4/1 -> loop breaker/1, To Workspace6/1
  Sum6/1 -> BS Logic/4(ECdiff1), To Workspace17/1
  ECPY (E')/1 -> To Workspace1/1, Sum6/2, Transport Delay9/1, OMN2/1(from NI)
  Transport Delay10/1 -> Sum4/1
  Transport Delay9/1 -> Sum4/2
  loop breaker/1 -> IM Sacc out/1

== system cnlib/CN SP+Sacc +BS (5/4)/OMN2 ==
  note: OMN
  note: Note that the OMN properly combines the pulse with the output of the NI, by latching
      | that output to its value at the moment the pulse appears.
  note: Operation: when the pulse is active ("from PG") it activates the switch, passing the
      | upper input through to the output.  When the pulse is over, the switch changes,
      | allowing the lower input (from the NI) to pass.
  note: This block behaves like the ocular motor neurons,combining a phasic pulse (from PG)
      | with the tonic step produced by integration of the step, yielding a Pulse-Step
      | to drive the plant.
  from NI : Inport  Port=1  LatchInput=off
  from PG : Inport  Port=2  LatchInput=off
  Abs : Abs  SaturateOnIntegerOverflow=on
  Gain _ : Gain  Gain=1.0  SaturateOnIntegerOverflow=on
  SampHold? : Subsystem
      mask Display: disp('S&H\n(L)')
  Sign : Subsystem
      mask Type: Sign
      mask Description: y = sign(x)
      mask Help: Sign Function:\n\t\t\ty = 1 if x > 0\n\t\t\ty = 0 if x = 0\n\t\t\ty = -1 if x < 0
      mask Display: plot(-50,-50,50,50,[-50,50],[0,0],[0,0],[-50,50],[-40,0],[-30,-30],[0,40],[30,30])
  Sum : Sum  SaturateOnIntegerOverflow=on  InputSameDT=on
  Switch : Switch  Threshold=.5  SaturateOnIntegerOverflow=on  InputSameDT=on
  out_1 : Outport  InitialOutput=0
  wires:
  from NI/1 -> Switch/3, SampHold?/1(Input)
  Sign/1(out_1) -> Switch/2, SampHold?/2(S/H?)
  Gain _/1 -> Sum/1
  SampHold?/1(output) -> Sum/2
  Sum/1 -> Switch/1
  from PG/1 -> Abs/1, Gain _/1
  Switch/1 -> out_1/1
  Abs/1 -> Sign/1(in_1)

== system cnlib/CN SP+Sacc +BS (5/4)/PG (simp) w/SH,latch ==
  note: While perhaps not physiological, it has the virtue of actually working
      | 1) predictably and 2) correctly, making it useful for testing of the rest of the model.
  note: It is also capable of generating saccades to the left or the right, and has a piece-wise
      | linear relationship for pulse width (for saccades >1 deg and those <1 degree).
  note: This is a somewhat simplified Pulse Generator.  It does not use feedback, as does the
      | original version, but rather uses the calculated PW and PH functions to deliver
      | a timed pulse of the specified magnitude.
  note: PG (simp) w/SH, Latch
  note: (Init input:1)
  note: (Init input:0)
  in_1 : Inport  Port=1  LatchInput=off
  Abs : Abs  SaturateOnIntegerOverflow=on
  Constant : Constant  Value=0
  MATLAB Fcn : MATLABFcn  MATLABFcn=PWsimp
      mask Help: u>=1: y=(1.3*abs(u)+12)/1000\nu <1: y=(12*abs(u))/1000
      mask Display: disp('PW\nsimp')
  MATLAB Fcn1 : MATLABFcn  MATLABFcn=PHsimp
      mask Help: u<=0.25: y=0\nu> 0.25:  y = 590*u/(7.5+abs(u))
      mask Display: disp('PH\nsimp')
  RefLatch (good) : Subsystem  Orientation=left  mask{@1=50}
      mask prompts: @1 "Refractory Period (ms)"
      mask help: Refractory Latch
      mask init:
      | delay=@1;
      mask Display: disp('Refract\nLatch')
  SampHold?1 : Subsystem
      mask Display: disp('S&H\n(S=H)\n(H=L)')
  Sum : Sum  Inputs=+-  SaturateOnIntegerOverflow=on  InputSameDT=on
  Switch : Switch  Threshold=0.5  SaturateOnIntegerOverflow=on  InputSameDT=on
  To Workspace : ToWorkspace  VariableName=peakval  SaveFormat=Array
      settings: MaxDataPoints=10000
  To Workspace1 : ToWorkspace  VariableName=dur  SaveFormat=Array
      settings: MaxDataPoints=10000
  To Workspace2 : ToWorkspace  VariableName=pgtp1  SaveFormat=Array
      settings: MaxDataPoints=10000
  To Workspace3 : ToWorkspace  VariableName=shout  SaveFormat=Array
      settings: MaxDataPoints=10000
  To Workspace5 : ToWorkspace  VariableName=shin  SaveFormat=Array
      settings: MaxDataPoints=10000
  Variable Transport Delay : VariableTransportDelay  MaximumDelay=10  InitialInput=1
  loop breaker : Memory  Orientation=left
  out_1 : Outport  InitialOutput=0
  wires:
  MATLAB Fcn/1 -> Variable Transport Delay/2, To Workspace1/1
  Sum/1 -> Abs/1
  Abs/1 -> Switch/2
  loop breaker/1 -> RefLatch (good)/1(in_1)
  Variable Transport Delay/1 -> To Workspace2/1, Sum/2
  Constant/1 -> Switch/3
  Switch/1 -> loop breaker/1, out_1/1
  MATLAB Fcn1/1 -> Switch/1, Variable Transport Delay/1, Sum/1, To Workspace/1
  in_1/1 -> SampHold?1/1(Input), To Workspace5/1
  SampHold?1/1(output) -> MATLAB Fcn1/1, MATLAB Fcn/1, To Workspace3/1
  RefLatch (good)/1(out_1) -> SampHold?1/2(S/H?)

== system cnlib/CN SP+Sacc +BS (5/4)/lead/trail edge det 1 ==
  note: leading/trailing edge detection
  in_1 : Inport  Port=1  LatchInput=off
  Abs2 : Abs  SaturateOnIntegerOverflow=on
  Constant5 : Constant  Orientation=up  Value=0.0
  Constant6 : Constant  Orientation=down  Value=1.0
  Derivative2 : Derivative
  Switch2 : Switch  Threshold=150  SaturateOnIntegerOverflow=on  InputSameDT=on
  out_1 : Outport  InitialOutput=0
  wires:
  Constant6/1 -> Switch2/1
  Abs2/1 -> Switch2/2
  Derivative2/1 -> Abs2/1
  in_1/1 -> Derivative2/1
  Switch2/1 -> out_1/1
  Constant5/1 -> Switch2/3
